simulink model "explicit_test"  (R2024a)
settings: Solver=FixedStepAuto  StartTime=0.0  StopTime=10.0  FixedStep=0.05  RelTol=1e-3
PostLoadFcn:
  | on_model_load
StartFcn:
  | on_model_start
StopFcn:
  | on_simulation_done
undefined symbols (not defined in the file or in its folder): ActiveScenario
libraries: data_driven_lib_ctl x2, mss_wrappers x2, SignalEditorBlockLib x1
PostSaveFcn:
  | on_model_save
settings Model: Creator=luka  LastModifiedBy=luka

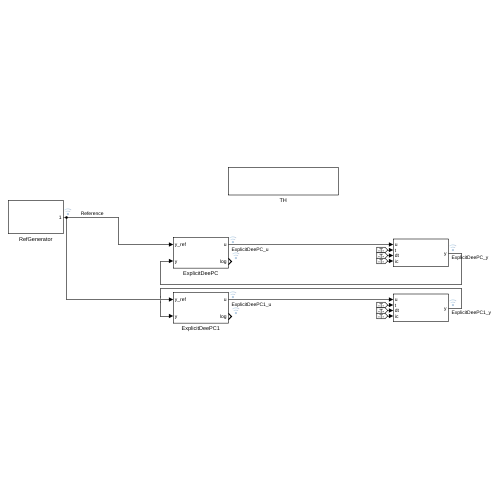
[thumbnail: Simulink's stored preview of the top-level diagram]
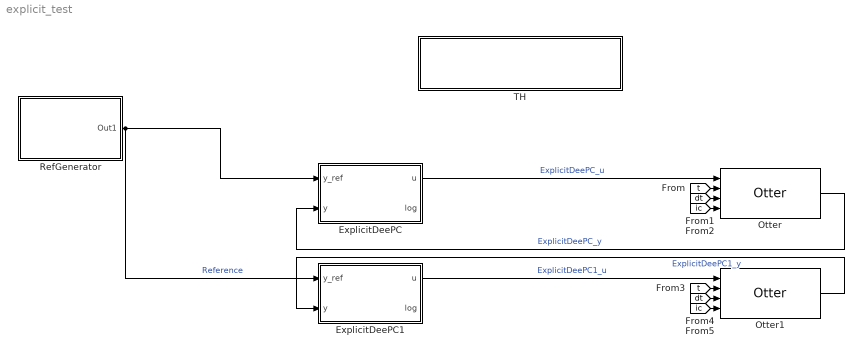
== system explicit_test ==
  ExplicitDeePC : Subsystem
  ExplicitDeePC1 : Subsystem
  Otter : mss_wrappers/Otter  Tag=system;__cs_slx_sys;  params=Otter_params  merged_params=ActiveScenario.Params
  Otter1 : mss_wrappers/Otter  Tag=system;__cs_slx_sys;  params=Otter_params  merged_params=ActiveScenario.Params
  RefGenerator : Subsystem  mask{scenario=P1}
      settings: OpenFcn=on_reference_generator_open();
      mask TypeOptions scenario: P1
      mask Callback scenario: on_reference_select;
      mask DialogControl edit_refs_btn Prompt: Edit references
      mask DialogControl edit_refs_btn Callback: on_edit_references_btn;
  TH : Subsystem
      mask DialogControl ParameterGroupVar Prompt: Params
  wires:
  [t] -> Otter/2
  [dt] -> Otter/3
  [ic] -> Otter/4
  [t] -> Otter1/2
  [dt] -> Otter1/3
  [ic] -> Otter1/4
  ExplicitDeePC/1(u) -> Otter/1  "ExplicitDeePC_u"
  Otter/1 -> ExplicitDeePC/2(y)  "ExplicitDeePC_y"
  RefGenerator/1(Out1) -> ExplicitDeePC/1(y_ref), ExplicitDeePC1/1(y_ref)  "Reference"
  ExplicitDeePC1/1(u) -> Otter1/1  "ExplicitDeePC1_u"
  Otter1/1 -> ExplicitDeePC1/2(y)  "ExplicitDeePC1_y"

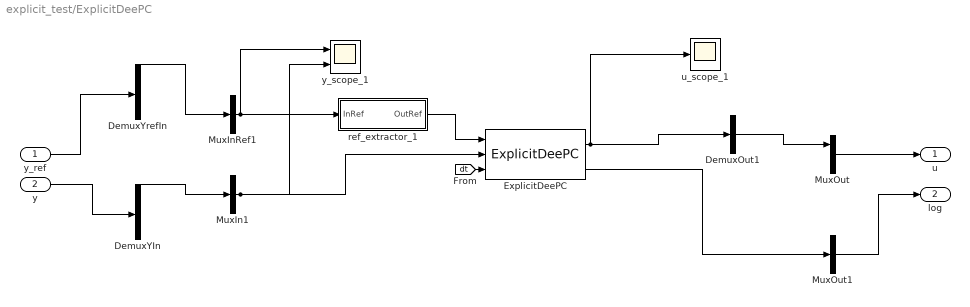
== system explicit_test/ExplicitDeePC ==
  y_ref : Inport  PortDimensions=12
  y : Inport  Port=2  PortDimensions=12
  DemuxOut1 : Demux  Outputs=1
  DemuxYIn : Demux  Outputs=12
  DemuxYrefIn : Demux  Outputs=12
  ExplicitDeePC : data_driven_lib_ctl/ExplicitDeePC  Tag=__cs_m_ctl;  params=explicit_params2  data=ExplicitDeePC_data  ParamsType=ExplicitDeePC_PT  DataType=ExplicitDeePC_DT  LogEntryType=ExplicitDeePC_LT  u_ic=0
  MuxIn1 : Mux  Inputs=1
  MuxInRef1 : Mux  Inputs=1
  MuxOut : Mux  Inputs=2
  MuxOut1 : BusCreator  Inputs=1
  ref_extractor_1 : Subsystem
  u_scope_1 : Scope
  y_scope_1 : Scope  NumInputPorts=2
  u : Outport  PortDimensions=2
  log : Outport  Port=2
  wires:
  [dt] -> ExplicitDeePC/3
  y/1 -> DemuxYIn/1
  y_ref/1 -> DemuxYrefIn/1
  MuxOut/1 -> u/1
  MuxOut1/1 -> log/1
  MuxInRef1/1 -> ref_extractor_1/1(InRef), y_scope_1/1
  ref_extractor_1/1(OutRef) -> ExplicitDeePC/1
  MuxIn1/1 -> ExplicitDeePC/2, y_scope_1/2
  ExplicitDeePC/1 -> DemuxOut1/1, u_scope_1/1
  ExplicitDeePC/2 -> MuxOut1/1
  DemuxYIn/1 -> MuxIn1/1
  DemuxYrefIn/1 -> MuxInRef1/1
  DemuxOut1/1 -> MuxOut/1

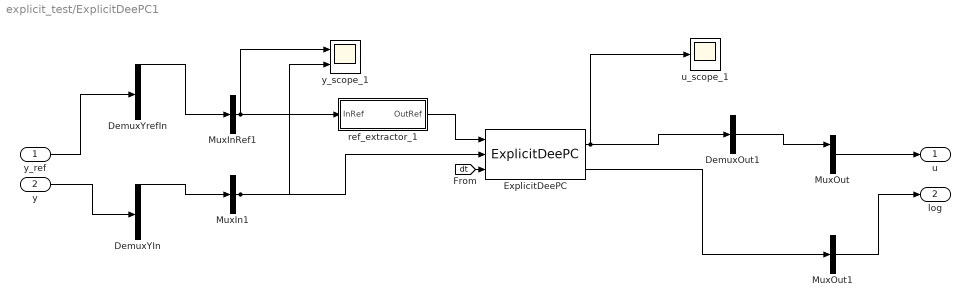
== system explicit_test/ExplicitDeePC1 ==
  y_ref : Inport  PortDimensions=12
  y : Inport  Port=2  PortDimensions=12
  DemuxOut1 : Demux  Outputs=1
  DemuxYIn : Demux  Outputs=12
  DemuxYrefIn : Demux  Outputs=12
  ExplicitDeePC : data_driven_lib_ctl/ExplicitDeePC  Tag=__cs_m_ctl;  params=explicit_params  data=ExplicitDeePC_data  ParamsType=ExplicitDeePC_PT  DataType=ExplicitDeePC_DT  LogEntryType=ExplicitDeePC_LT  u_ic=0
  MuxIn1 : Mux  Inputs=1
  MuxInRef1 : Mux  Inputs=1
  MuxOut : Mux  Inputs=2
  MuxOut1 : BusCreator  Inputs=1
  ref_extractor_1 : Subsystem
  u_scope_1 : Scope
  y_scope_1 : Scope  NumInputPorts=2
  u : Outport  PortDimensions=2
  log : Outport  Port=2
  wires:
  [dt] -> ExplicitDeePC/3
  y/1 -> DemuxYIn/1
  y_ref/1 -> DemuxYrefIn/1
  MuxOut/1 -> u/1
  MuxOut1/1 -> log/1
  MuxInRef1/1 -> ref_extractor_1/1(InRef), y_scope_1/1
  ref_extractor_1/1(OutRef) -> ExplicitDeePC/1
  MuxIn1/1 -> ExplicitDeePC/2, y_scope_1/2
  ExplicitDeePC/1 -> DemuxOut1/1, u_scope_1/1
  ExplicitDeePC/2 -> MuxOut1/1
  DemuxYIn/1 -> MuxIn1/1
  DemuxYrefIn/1 -> MuxInRef1/1
  DemuxOut1/1 -> MuxOut/1

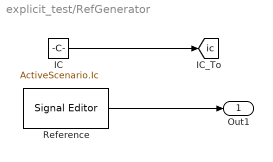
== system explicit_test/RefGenerator ==
  IC : Constant  Value=ActiveScenario.Ic
  Reference : SignalEditorBlockLib/Signal Editor  FileName=untitled.mat  ActiveScenario=Scenario  ActiveSignal=Signal 1  IsBus=off  OutputBusObjectStr=Bus: BusObject  SampleTime=0  Interpolate=off  ZeroCross=off  OutputAfterFinalValue=Setting to zero  Unit=inherit  PreserveSignalName=on  ApplySigPropsToAllScenarios=on  ApplySigPropsToAllSignals=off
  Out1 : Outport
  tag scope: ic=global
  wires:
  IC/1 -> [ic]
  Reference/1 -> Out1/1

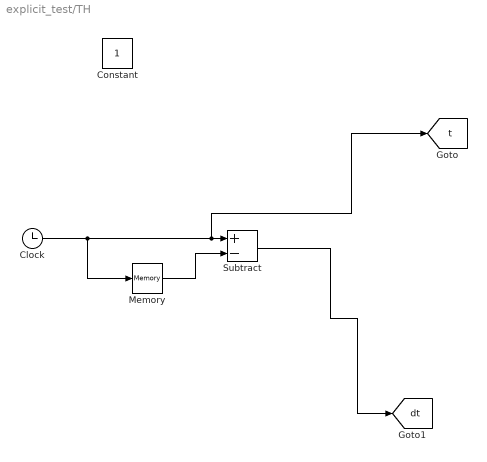
== system explicit_test/TH ==
  Clock : Clock
  Constant : Constant
  Memory : Memory
  Subtract : Sum  Inputs=+-
  tag scope: dt=global, t=global
  wires:
  Subtract/1 -> [dt]
  Memory/1 -> Subtract/2
  Clock/1 -> Memory/1, Subtract/1, [t]

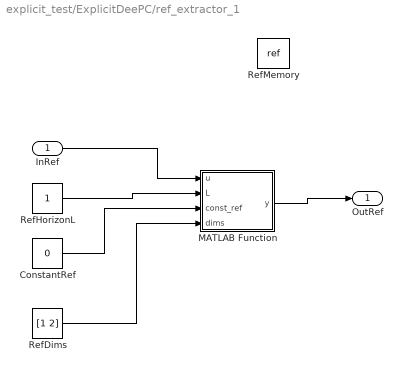
== system explicit_test/ExplicitDeePC/ref_extractor_1 ==
  InRef : Inport
  ConstantRef : Constant  Value=0
  MATLAB Function : MATLAB Function  TreatAsAtomicUnit=on
  RefDims : Constant  Value=[1 2]
  RefHorizonL : Constant
  RefMemory : DataStoreMemory  DataStoreName=ref  WriteAfterWriteMsg=warning  ShowAdditionalParam=off  OutDataTypeStr=double
  OutRef : Outport
  wires:
  ConstantRef/1 -> MATLAB Function/3(const_ref)
  RefDims/1 -> MATLAB Function/4(dims)
  RefHorizonL/1 -> MATLAB Function/2(L)
  InRef/1 -> MATLAB Function/1(u)
  MATLAB Function/1(y) -> OutRef/1

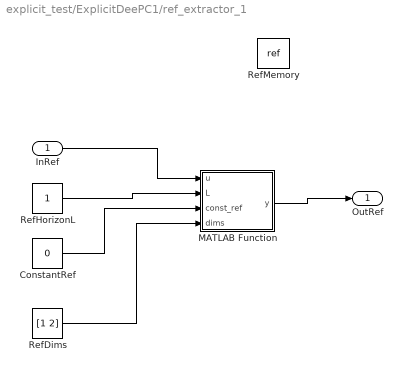
== system explicit_test/ExplicitDeePC1/ref_extractor_1 ==
  InRef : Inport
  ConstantRef : Constant  Value=0
  MATLAB Function : MATLAB Function  TreatAsAtomicUnit=on
  RefDims : Constant  Value=[1 2]
  RefHorizonL : Constant
  RefMemory : DataStoreMemory  DataStoreName=ref  WriteAfterWriteMsg=warning  ShowAdditionalParam=off  OutDataTypeStr=double
  OutRef : Outport
  wires:
  ConstantRef/1 -> MATLAB Function/3(const_ref)
  RefDims/1 -> MATLAB Function/4(dims)
  RefHorizonL/1 -> MATLAB Function/2(L)
  InRef/1 -> MATLAB Function/1(u)
  MATLAB Function/1(y) -> OutRef/1

== matlab function explicit_test/ExplicitDeePC1/ref_extractor_1/MATLAB Function ==
  settings: updateMethod=DISCRETE
  data: u input; L input; const_ref input; dims input; y output; ref data_store_memory; GlobalReference parameter
function y = fcn(u, L, const_ref, dims, GlobalReference)

persistent cnt
global ref

if isempty(cnt)
    cnt = 0;
end
cnt = cnt+1;

horizon_end = cnt+L-1;
if L > 1 
   if horizon_end > length(GlobalReference)
        if size(ref, 1) == size(u, 1)
            y = permute(ref, [2, 1]);
        else
            y = ref;
        end       
        return
   end

   if size(ref, 1) == size(u, 1)
      
      if const_ref == 0
        ref(:, :) = GlobalReference(cnt:horizon_end, dims)';
      else
        ref(:, :) = repmat(GlobalReference(cnt, dims)', 1, L);
      end
      y = permute(ref, [2, 1]);
   else
      if const_ref == 0
        ref(1:L, :) = GlobalReference(cnt:horizon_end, dims);
      else
        ref(1:L, :) = repmat(GlobalReference(cnt, dims), L, 1);
      end
      y = ref;
   end
else
   if size(ref, 1) == size(u, 1)
       ref = u;
       y = permute(ref, [2, 1]);
   else
      ref(1, :) = u';
      y = ref;
   end
end

== matlab function explicit_test/ExplicitDeePC/ref_extractor_1/MATLAB Function ==
  settings: updateMethod=DISCRETE
  data: u input; L input; const_ref input; dims input; y output; ref data_store_memory; GlobalReference parameter
function y = fcn(u, L, const_ref, dims, GlobalReference)

persistent cnt
global ref

if isempty(cnt)
    cnt = 0;
end
cnt = cnt+1;

horizon_end = cnt+L-1;
if L > 1 
   if horizon_end > length(GlobalReference)
        if size(ref, 1) == size(u, 1)
            y = permute(ref, [2, 1]);
        else
            y = ref;
        end       
        return
   end

   if size(ref, 1) == size(u, 1)
      
      if const_ref == 0
        ref(:, :) = GlobalReference(cnt:horizon_end, dims)';
      else
        ref(:, :) = repmat(GlobalReference(cnt, dims)', 1, L);
      end
      y = permute(ref, [2, 1]);
   else
      if const_ref == 0
        ref(1:L, :) = GlobalReference(cnt:horizon_end, dims);
      else
        ref(1:L, :) = repmat(GlobalReference(cnt, dims), L, 1);
      end
      y = ref;
   end
else
   if size(ref, 1) == size(u, 1)
       ref = u;
       y = permute(ref, [2, 1]);
   else
      ref(1, :) = u';
      y = ref;
   end
end
